simulink model "SEA_system"  (R2023b)
settings: Solver=VariableStepAuto  StartTime=0.0  StopTime=10  FixedStep=0.005  RelTol=1e-3
values from neighbouring files (symbols this model uses):
  c1 = 0.6    [SEA_system.m]
  c2 = 0.6    [SEA_system.m]
  CoM1 = 0.117    [SEA_system.m]
  CoM2 = 0.045    [SEA_system.m]
  Fx = 0    [SEA_system.m]
  Fy = 0    [SEA_system.m]
  g = 9.81    [SEA_system.m]
  J1 = m1*L1^2/12 + m1*CoM1^2    (= 0.00579610927083)    [SEA_system.m]
  J2 = m2*L2^2/12 + m2*CoM2^2 + (mEE*(L2-CoM2)^2)    (= 0.00129963166667)    [SEA_system.m]
  k1 = 5.9*10^3    (= 5900)    [SEA_system.m]
  k2 = 5.9*10^3    (= 5900)    [SEA_system.m]
  L1 = 0.20075    [SEA_system.m]
  L2 = 0.149    [SEA_system.m]
  m1 = 0.340    (= 0.34)    [SEA_system.m]
  m2 = 0.140    (= 0.14)    [SEA_system.m]
  N1 = m1*CoM1^2 + J1 + m2*L1^2 + m2*CoM2^2 + J2    (= 0.0176755796875)    [SEA_system.m]
  N2 = m2*L1*CoM2    (= 0.001264725)    [SEA_system.m]
  N3 = m2*CoM2^2 + J2    (= 0.00158313166667)    [SEA_system.m]
  Px = 0.1    [SEA_system.m]
  Py = 0.05    [SEA_system.m]
libraries: simulink_extras x4, slpidlib x3
settings Model: Creator=Master  LastModifiedBy=tpdnr
settings SolverCC: ZeroCrossAlgorithm=Adaptive
settings DebuggingCC: MaskedZcDiagnostic=none  IgnoredZcDiagnostic=none

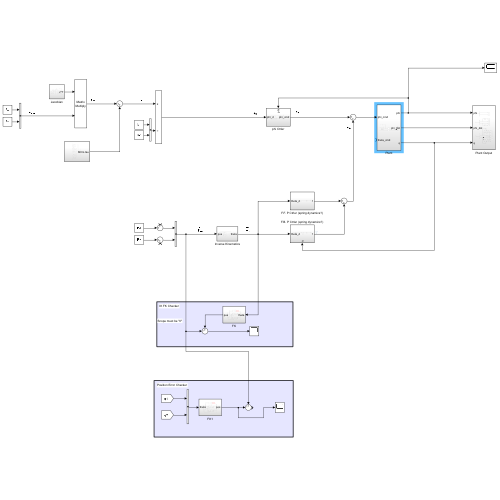
[thumbnail: Simulink's stored preview of the top-level diagram]
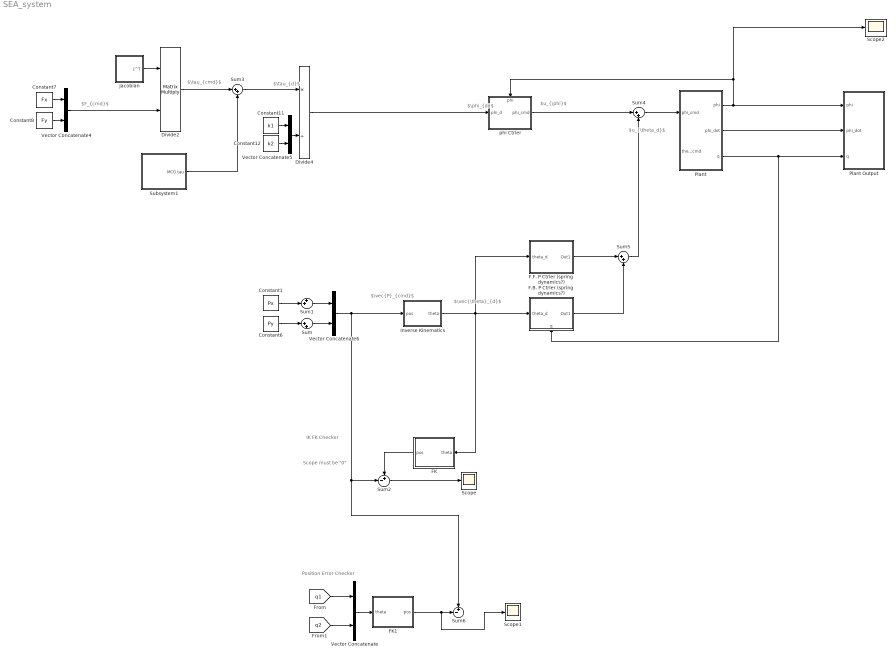
== system SEA_system ==
  note: Position Error Checker
  note: Scope must be "0"
  note: $F_{cmd}$
  note: $\tau_{cmd}$
  note: $\tau_{d}$
  note: $\phi_{d}$
  note: $u_{\phi}$
  note: $\vec{P}_{cmd}$
  note: $\vec{\theta}_{d}$
  note: $u_{\theta_d}$
  note: IK FK Checker
  Constant1 : Constant  Value=Px
  Constant11 : Constant  Value=k1
  Constant12 : Constant  Value=k2
  Constant6 : Constant  Value=Py
  Constant7 : Constant  Value=Fx
  Constant8 : Constant  Value=Fy
  Divide2 : Product  Inputs=**  Multiplication=Matrix(*)
  Divide4 : Product  Inputs=*/
  F.B. P Ctrler (spring dynamics?) : Subsystem
      settings: PortSchema="{\"entries\":[{\"content\":{\"sides\":[{\"content\":{\"connectorIds\":[\"In1\"]},\"type\":\"ConnectorPlacement.EquallySpacedRectSide\",\"uuid\":\"4d208e63-a6c3-42c2-9e85-ad51048c4a51\"},{\"content\":{\"connectorIds\":[\"Out1\"],\"side\":\"RIGHT\"},\"type\":\"ConnectorPlacement.EquallySpacedRectSide\",\"uuid\":\"eee0dd30-27df-41b3-9dcf-f04dc984317a\"},{\"content\":{\"side\":\"TOP\"},\"type\":\"ConnectorPlacement.EquallySpacedRectSide\",\"uuid\":\"b56dc6f1-fbae-4ae5-b685-d1dd5f7423cb\"},{\"content\":{\"connectorIds\":[\"In2\"],\"side\":\"BOTTOM\"},\"type\":\"ConnectorPlacement.EquallySpacedRectSide\",\"uuid\":\"8db1bbe8-a585-485d-a15a-1764a5483703\"}]},\"type\":\"ConnectorPlacement.EquallySpacedConnector\",\"uuid\":\"2ec91dce-e516-4ac5-924e-aa549dba9b81\"}],\"packageUris\":[\"http://schema.mathworks.com/mf0/Connector/R2020b\"],\"version\":\"1.0\"}"
  F.F. P Ctrler (spring dynamics?) : Subsystem
  FK : Subsystem
  FK1 : Subsystem
      settings: PortSchema="{\"entries\":[{\"content\":{\"sides\":[{\"content\":{\"connectorIds\":[\"Out1\"]},\"type\":\"ConnectorPlacement.EquallySpacedRectSide\",\"uuid\":\"9148f4d4-3f7b-4339-b598-70e7eba9c14c\"},{\"content\":{\"connectorIds\":[\"In1\"],\"side\":\"RIGHT\"},\"type\":\"ConnectorPlacement.EquallySpacedRectSide\",\"uuid\":\"2ec983d7-29f9-4bcc-b0b0-e28b197ebcd0\"},{\"content\":{\"side\":\"TOP\"},\"type\":\"ConnectorPlacement.EquallySpacedRectSide\",\"uuid\":\"6d95d5e6-a927-40b0-a022-88fc1901032f\"}]},\"type\":\"ConnectorPlacement.EquallySpacedConnector\",\"uuid\":\"4f8038e9-ada6-4d65-8522-250804851321\"}],\"packageUris\":[\"http://schema.mathworks.com/mf0/Connector/R2020b\"],\"version\":\"1.0\"}"
  Inverse Kinematics : Subsystem
  Jacobian : Subsystem
  Plant : Subsystem
  Plant Output : Subsystem
  Scope : Scope
  Scope1 : Scope
  Scope2 : Scope
  Subsystem1 : Subsystem
  Sum{,3..5} (4 alike) : Sum  Inputs=|++
  Sum1 : Sum  Inputs=++|
  Sum2 : Sum  Inputs=+-|
  Sum6 : Sum  Inputs=+-|
  Vector Concatenate{,4..6} (4 alike) : Concatenate
  phi Ctrler : Subsystem
      settings: PortSchema="{\"entries\":[{\"content\":{\"sides\":[{\"content\":{\"connectorIds\":[\"In1\"]},\"type\":\"ConnectorPlacement.EquallySpacedRectSide\",\"uuid\":\"3d32bdc1-b9b0-4014-9f2c-584152c2ae2a\"},{\"content\":{\"connectorIds\":[\"Out1\"],\"side\":\"RIGHT\"},\"type\":\"ConnectorPlacement.EquallySpacedRectSide\",\"uuid\":\"debc5263-adf8-4ed2-a891-d4f334c5857b\"},{\"content\":{\"connectorIds\":[\"In2\"],\"side\":\"TOP\"},\"type\":\"ConnectorPlacement.EquallySpacedRectSide\",\"uuid\":\"7bd5ab05-8083-45fb-a57a-66a3a725ceed\"}]},\"type\":\"ConnectorPlacement.EquallySpacedConnector\",\"uuid\":\"986cff17-d96f-4d8b-90f2-1c94d4d77448\"}],\"packageUris\":[\"http://schema.mathworks.com/mf0/Connector/R2020b\"],\"version\":\"1.0\"}"
  wires:
  Constant7/1 -> Vector Concatenate4/1
  Constant8/1 -> Vector Concatenate4/2
  Vector Concatenate5/1 -> Divide4/2
  Constant11/1 -> Vector Concatenate5/1
  Constant12/1 -> Vector Concatenate5/2
  Divide4/1 -> phi Ctrler/1(phi_d)
  Inverse Kinematics/1(theta) -> FK/1(theta), F.F. P Ctrler (spring dynamics?)/1(theta_d), F.B. P Ctrler (spring dynamics?)/1(theta_d)
  Plant/1(phi) -> Plant Output/1(phi), phi Ctrler/2(phi), Scope2/1
  Plant/3(q) -> F.B. P Ctrler (spring dynamics?)/2(q), Plant Output/3(q)
  Jacobian/1(J^T) -> Divide2/1
  Vector Concatenate4/1 -> Divide2/2
  Vector Concatenate6/1 -> Sum6/1, Sum2/2, Inverse Kinematics/1(pos)
  Sum5/1 -> Sum4/2
  phi Ctrler/1(phi_cmd) -> Sum4/1
  Constant1/1 -> Sum1/2
  Constant6/1 -> Sum/1
  Sum/1 -> Vector Concatenate6/2
  Sum1/1 -> Vector Concatenate6/1
  FK/1(pos) -> Sum2/1
  [q1] -> Vector Concatenate/1
  [q2] -> Vector Concatenate/2
  Vector Concatenate/1 -> FK1/1(theta)
  F.F. P Ctrler (spring dynamics?)/1(Out1) -> Sum5/1
  F.B. P Ctrler (spring dynamics?)/1(Out1) -> Sum5/2
  Sum2/1 -> Scope/1
  FK1/1(pos) -> Scope1/1, Sum6/2
  Plant/2(phi_dot) -> Plant Output/2(phi_dot)
  Divide2/1 -> Sum3/1
  Subsystem1/1(MCG tau) -> Sum3/2
  Sum3/1 -> Divide4/1
  Sum4/1 -> Plant/1(phi_cmd)

== system SEA_system/F.B. P Ctrler (spring dynamics?) ==
  note: $e_{\theta}$
  note: $Controller$
  theta_d : Inport
  q : Inport  Port=2
  Gain : Gain
  PID Controller : slpidlib/PID Controller  Controller=PID  Form=Parallel  TimeDomain=Continuous-time  UseExternalTs=off  SampleTime=-1  IntegratorMethod=Forward Euler  FilterMethod=Forward Euler  ControllerParametersSource=internal  P=10  I=1  UseKiTs=off  D=0  N=100  UseFilter=on  TunerSelectOption=Transfer Function Based (PID Tuner App)  InitialConditionSource=internal  InitialConditionForIntegrator=0  InitialConditionForFilter=0  DifferentiatorICPrevScaledInput=0  ExternalReset=none  TrackingMode=off  Kt=1  LimitOutput=off  SatLimitsSource=internal  UpperSaturationLimit=inf  LowerSaturationLimit=-inf  LinearizeAsGain=on  AntiWindupMode=none  Kb=1  LimitIntegrator=off  UpperIntegratorSaturationLimit=inf  LowerIntegratorSaturationLimit=-inf  POutMin=[]  POutMax=[]  IOutMin=[]  IOutMax=[]  DOutMin=[]  DOutMax=[]  NOutMin=[]  NOutMax=[]  SumOutMin=[]  SumOutMax=[]  SaturationOutMin=[]  SaturationOutMax=[]  PParamMin=[]  PParamMax=[]  IParamMin=[]  IParamMax=[]  DParamMin=[]  DParamMax=[]  NParamMin=[]  NParamMax=[]  KbParamMin=[]  KbParamMax=[]  KtParamMin=[]  KtParamMax=[]  KbOutMin=[]  KbOutMax=[]  KtOutMin=[]  KtOutMax=[]  IntegratorOutMin=[]  IntegratorOutMax=[]  FilterOutMin=[]  FilterOutMax=[]  SumI1OutMin=[]  SumI1OutMax=[]  SumI2OutMin=[]  SumI2OutMax=[]  SumI3OutMin=[]  SumI3OutMax=[]  SumI4OutMin=[]  SumI4OutMax=[]  SumDOutMin=[]  SumDOutMax=[]  DifferentiatorOutMin=[]  DifferentiatorOutMax=[]  FilterDiffOutCoefMin=[]  FilterDiffOutCoefMax=[]  ReciprocalOutMin=[]  ReciprocalOutMax=[]  SumDenOutMin=[]  SumDenOutMax=[]  SumNumOutMin=[]  SumNumOutMax=[]  DivideOutMin=[]  DivideOutMax=[]  UdiffTsProdOutMin=[]  UdiffTsProdOutMax=[]  NTsProdOutMin=[]  NTsProdOutMax=[]  UintegralTsProdOutMin=[]  UintegralTsProdOutMax=[]  UngainTsProdOutMin=[]  UngainTsProdOutMax=[]  ClampingZeroOutDataTypeStr=Inherit: Inherit via back propagation  ClampingZeroOutMin=[]  ClampingZeroOutMax=[]  FilterDenConstantOutDataTypeStr=Inherit: Inherit via back propagation  FilterDenConstantOutMin=[]  FilterDenConstantOutMax=[]  PCopyOutDataTypeStr=Inherit: Inherit via back propagation  PCopyOutMin=[]  PCopyOutMax=[]  NCopyOutDataTypeStr=Inherit: Inherit via back propagation  NCopyOutMin=[]  NCopyOutMax=[]  IntegratorContinuousStateAttributes=''  IntegratorStateMustResolveToSignalObject=off  IntegratorRTWStateStorageClass=Auto  FilterContinuousStateAttributes=''  FilterStateMustResolveToSignalObject=off  FilterRTWStateStorageClass=Auto  ParallelPVariant=InternalParameters  IdealPVariant=Disabled  IVariant=InternalParameters  DVariant=InternalParameters  IntegratorVariant=Continuous  SatVariant=Disabled  AWVariant=Passthrough  PCopyVariant=Disabled  TRVariant=Disabled  FdbkBlocksVariant=Forward  IdealPFdbkVariant=Disabled  SatFdbkVariant=Disabled  DerivativeFilterVariant=ContFilter  NVariant=InternalParameters  NCopyVariant=Disabled  FilterICVariant=InternalICsFilter  IntegratorICVariant=InternalICs  ExternalResetVariant=Disabled  TRSumVariant=Passthrough  SumFdbkVariant=Disabled  SumVariant=Sum_PID  TsampFilterVariant=InternalTs  TsampNgainVariant=Passthrough  TsampIntegralVariant=Disabled_SignalSpec  ExternalSaturationOutDataTypeStr=Inherit: Same as second input
  Sum : Sum  Inputs=|+-
  Out1 : Outport
  wires:
  Gain/1 -> Out1/1
  theta_d/1 -> Sum/1
  q/1 -> Sum/2
  Sum/1 -> PID Controller/1
  PID Controller/1 -> Gain/1

== system SEA_system/F.F. P Ctrler (spring dynamics?) ==
  note: $Controller$
  theta_d : Inport
  Gain : Gain
  Out1 : Outport
  wires:
  Gain/1 -> Out1/1
  theta_d/1 -> Gain/1

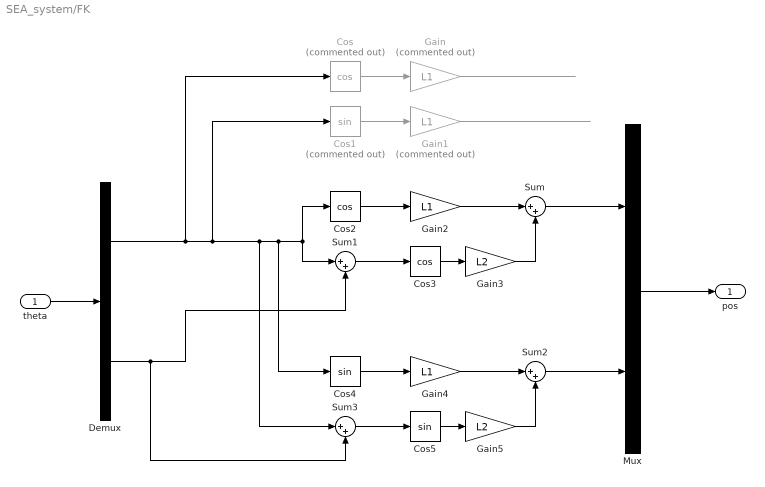
== system SEA_system/FK ==
  theta : Inport
  Cos : Trigonometry  Commented=on  Operator=cos
  Cos1 : Trigonometry  Commented=on
  Cos2 : Trigonometry  Operator=cos
  Cos3 : Trigonometry  Operator=cos
  Cos4 : Trigonometry
  Cos5 : Trigonometry
  Demux : Demux  Outputs=2
  Gain : Gain  Commented=on  Gain=L1
  Gain1 : Gain  Commented=on  Gain=L1
  Gain2 : Gain  Gain=L1
  Gain3 : Gain  Gain=L2
  Gain4 : Gain  Gain=L1
  Gain5 : Gain  Gain=L2
  Mux : Mux  Inputs=2
  Sum{,1..3} (4 alike) : Sum  Inputs=|++
  pos : Outport
  wires:
  Cos2/1 -> Gain2/1
  Cos3/1 -> Gain3/1
  Demux/1 -> Cos/1, Cos1/1, Sum3/1, Cos4/1, Cos2/1, Sum1/1
  Sum/1 -> Mux/1
  Demux/2 -> Sum3/2, Sum1/2
  Cos1/1 -> Gain1/1
  Cos5/1 -> Gain5/1
  Gain2/1 -> Sum/1
  Gain1/1 -> ?
  Cos/1 -> Gain/1
  Sum2/1 -> Mux/2
  Gain4/1 -> Sum2/1
  theta/1 -> Demux/1
  Gain3/1 -> Sum/2
  Sum3/1 -> Cos5/1
  Gain5/1 -> Sum2/2
  Sum1/1 -> Cos3/1
  Cos4/1 -> Gain4/1
  Gain/1 -> ?
  Mux/1 -> pos/1

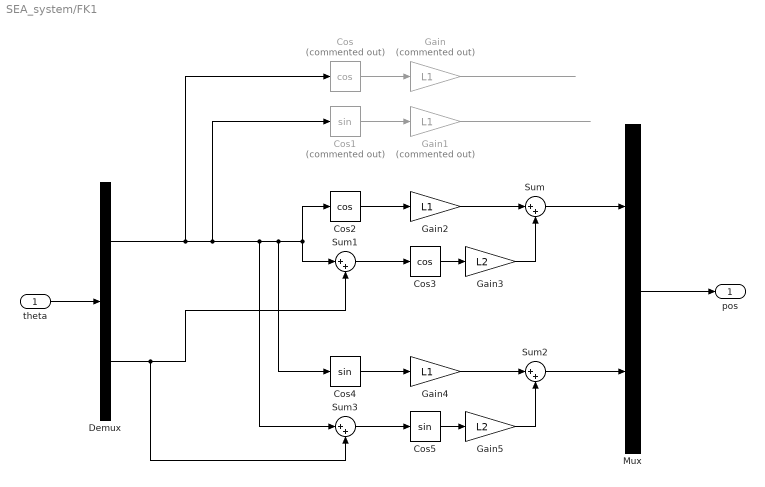
== system SEA_system/FK1 ==
  theta : Inport
  Cos : Trigonometry  Commented=on  Operator=cos
  Cos1 : Trigonometry  Commented=on
  Cos2 : Trigonometry  Operator=cos
  Cos3 : Trigonometry  Operator=cos
  Cos4 : Trigonometry
  Cos5 : Trigonometry
  Demux : Demux  Outputs=2
  Gain : Gain  Commented=on  Gain=L1
  Gain1 : Gain  Commented=on  Gain=L1
  Gain2 : Gain  Gain=L1
  Gain3 : Gain  Gain=L2
  Gain4 : Gain  Gain=L1
  Gain5 : Gain  Gain=L2
  Mux : Mux  Inputs=2
  Sum{,1..3} (4 alike) : Sum  Inputs=|++
  pos : Outport
  wires:
  Cos2/1 -> Gain2/1
  Cos3/1 -> Gain3/1
  Demux/1 -> Cos/1, Cos1/1, Sum3/1, Cos4/1, Cos2/1, Sum1/1
  Sum/1 -> Mux/1
  Demux/2 -> Sum3/2, Sum1/2
  Cos1/1 -> Gain1/1
  Cos5/1 -> Gain5/1
  Gain2/1 -> Sum/1
  Gain1/1 -> ?
  Cos/1 -> Gain/1
  Sum2/1 -> Mux/2
  Gain4/1 -> Sum2/1
  theta/1 -> Demux/1
  Gain3/1 -> Sum/2
  Sum3/1 -> Cos5/1
  Gain5/1 -> Sum2/2
  Sum1/1 -> Cos3/1
  Cos4/1 -> Gain4/1
  Gain/1 -> ?
  Mux/1 -> pos/1

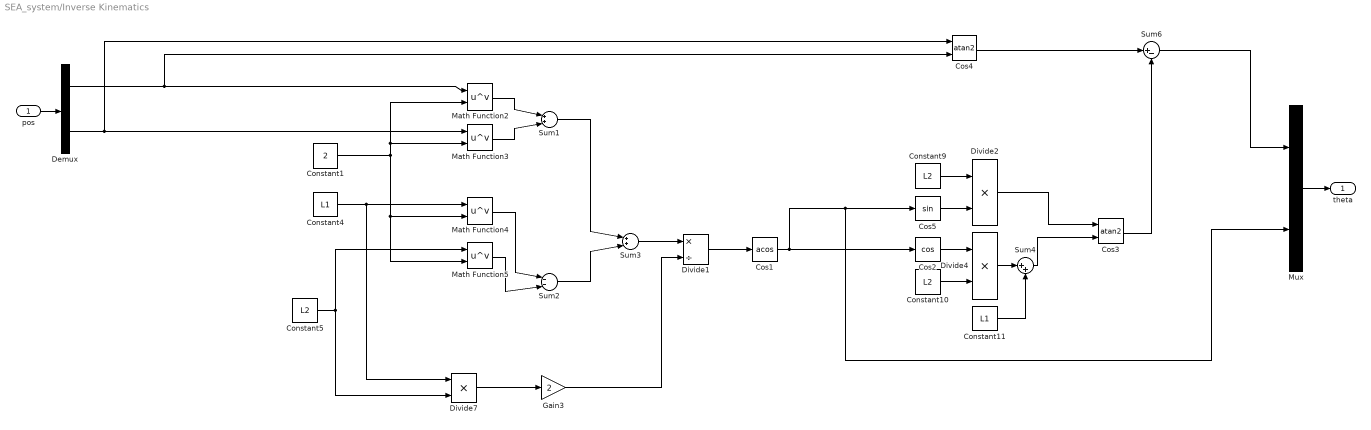
== system SEA_system/Inverse Kinematics ==
  pos : Inport
  Constant1 : Constant  Value=2
  Constant10 : Constant  Value=L2
  Constant11 : Constant  Value=L1
  Constant4 : Constant  Value=L1
  Constant5 : Constant  Value=L2
  Constant9 : Constant  Value=L2
  Cos1 : Trigonometry  Operator=acos
  Cos2 : Trigonometry  Operator=cos
  Cos3 : Trigonometry  Operator=atan2
  Cos4 : Trigonometry  Operator=atan2
  Cos5 : Trigonometry
  Demux : Demux  Outputs=2
  Divide1 : Product  Inputs=*/
  Divide2 : Product  Inputs=**
  Divide4 : Product  Inputs=**
  Divide7 : Product  Inputs=**
  Gain3 : Gain  Gain=2
  Math Function{2..5} (4 alike) : Math  Operator=pow
  Mux : Mux  Inputs=2
  Sum1 : Sum  Inputs=|++|
  Sum2 : Sum  Inputs=|--|
  Sum3 : Sum  Inputs=|++|
  Sum4 : Sum  Inputs=|++
  Sum6 : Sum  Inputs=|+-
  theta : Outport
  wires:
  Sum4/1 -> Cos3/2
  Cos3/1 -> Sum6/2
  Demux/1 -> Cos4/2, Math Function2/1
  Constant1/1 -> Math Function3/2, Math Function2/2, Math Function5/2, Math Function4/2
  Sum3/1 -> Divide1/1
  Constant5/1 -> Math Function5/1, Divide7/2
  Math Function4/1 -> Sum2/1
  Demux/2 -> Cos4/1, Math Function3/1
  Constant4/1 -> Divide7/1, Math Function4/1
  Gain3/1 -> Divide1/2
  Cos1/1 -> Mux/2, Cos5/1, Cos2/1
  Math Function3/1 -> Sum1/2
  Cos5/1 -> Divide2/2
  Constant10/1 -> Divide4/2
  Divide1/1 -> Cos1/1
  Sum1/1 -> Sum3/1
  Constant11/1 -> Sum4/2
  Math Function2/1 -> Sum1/1
  Constant9/1 -> Divide2/1
  Math Function5/1 -> Sum2/2
  Cos2/1 -> Divide4/1
  Cos4/1 -> Sum6/1
  Sum2/1 -> Sum3/2
  Divide7/1 -> Gain3/1
  Divide4/1 -> Sum4/1
  pos/1 -> Demux/1
  Mux/1 -> theta/1
  Divide2/1 -> Cos3/1
  Sum6/1 -> Mux/1

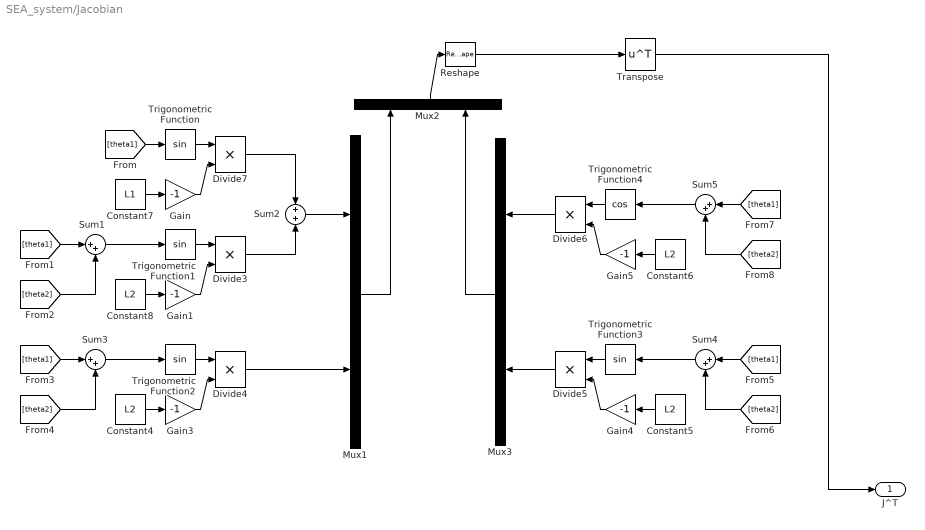
== system SEA_system/Jacobian ==
  Constant{4..6,8} (4 alike) : Constant  Value=L2
  Constant7 : Constant  Value=L1
  Divide{3..7} (5 alike) : Product  Inputs=**
  Gain{,1,3..5} (5 alike) : Gain  Gain=-1
  Mux1 : Mux  Inputs=2
  Mux2 : Mux  Inputs=2
  Mux3 : Mux  Inputs=2
  Reshape : Reshape  OutputDimensionality=Customize  OutputDimensions=[2,2]
  Sum{1,3..5} (4 alike) : Sum  Inputs=|++
  Sum2 : Sum  Inputs=+|+
  Transpose : Math  Operator=transpose
  Trigonometric Function{,1..3} (4 alike) : Trigonometry
  Trigonometric Function4 : Trigonometry  Operator=cos
  J^T : Outport
  wires:
  Gain1/1 -> Divide3/2
  [theta1] -> Sum5/1
  [theta1] -> Trigonometric Function/1
  Trigonometric Function4/1 -> Divide6/1
  Constant8/1 -> Gain1/1
  Mux2/1 -> Reshape/1
  Gain/1 -> Divide7/2
  [theta1] -> Sum4/1
  Constant5/1 -> Gain4/1
  [theta2] -> Sum1/2
  Sum4/1 -> Trigonometric Function3/1
  [theta2] -> Sum5/2
  Constant4/1 -> Gain3/1
  Trigonometric Function2/1 -> Divide4/1
  Divide3/1 -> Sum2/2
  Gain3/1 -> Divide4/2
  Mux1/1 -> Mux2/1
  Gain5/1 -> Divide6/2
  Trigonometric Function/1 -> Divide7/1
  Divide7/1 -> Sum2/1
  Trigonometric Function3/1 -> Divide5/1
  Sum3/1 -> Trigonometric Function2/1
  Sum5/1 -> Trigonometric Function4/1
  Trigonometric Function1/1 -> Divide3/1
  [theta1] -> Sum1/1
  Constant6/1 -> Gain5/1
  [theta2] -> Sum4/2
  Constant7/1 -> Gain/1
  Divide6/1 -> Mux3/1
  Mux3/1 -> Mux2/2
  [theta1] -> Sum3/1
  [theta2] -> Sum3/2
  Sum2/1 -> Mux1/1
  Sum1/1 -> Trigonometric Function1/1
  Gain4/1 -> Divide5/2
  Divide4/1 -> Mux1/2
  Divide5/1 -> Mux3/2
  Reshape/1 -> Transpose/1
  Transpose/1 -> J^T/1

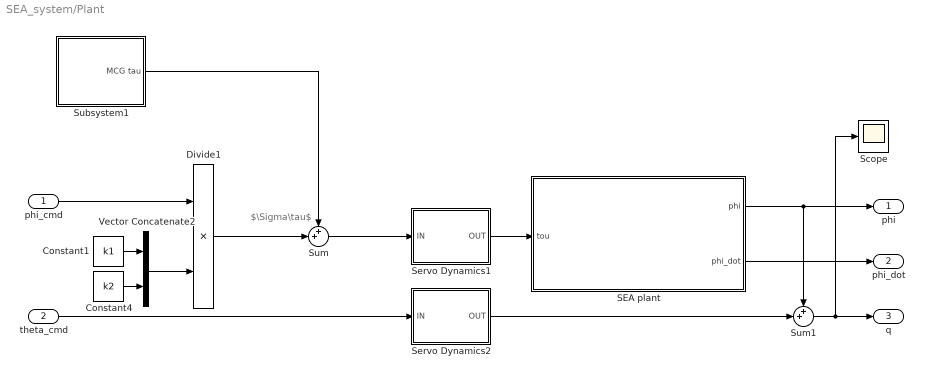
== system SEA_system/Plant ==
  note: $\Sigma\tau$
  phi_cmd : Inport
  theta_cmd : Inport  Port=2
  Constant1 : Constant  Value=k1
  Constant4 : Constant  Value=k2
  Divide1 : Product  Inputs=**
  SEA plant : Subsystem
  Scope : Scope
  Servo Dynamics1 : Subsystem
  Servo Dynamics2 : Subsystem
  Subsystem1 : Subsystem
  Sum : Sum  Inputs=++|
  Sum1 : Sum  Inputs=++|
  Vector Concatenate2 : Concatenate
  phi : Outport
  phi_dot : Outport  Port=2
  q : Outport  Port=3
  wires:
  SEA plant/1(phi) -> Sum1/1, phi/1
  Sum1/1 -> Scope/1, q/1
  Constant4/1 -> Vector Concatenate2/2
  Constant1/1 -> Vector Concatenate2/1
  Vector Concatenate2/1 -> Divide1/2
  phi_cmd/1 -> Divide1/1
  Servo Dynamics2/1(OUT) -> Sum1/2
  Servo Dynamics1/1(OUT) -> SEA plant/1(tou)
  SEA plant/2(phi_dot) -> phi_dot/1
  Subsystem1/1(MCG tau) -> Sum/1
  Sum/1 -> Servo Dynamics1/1(IN)
  theta_cmd/1 -> Servo Dynamics2/1(IN)
  Divide1/1 -> Sum/2

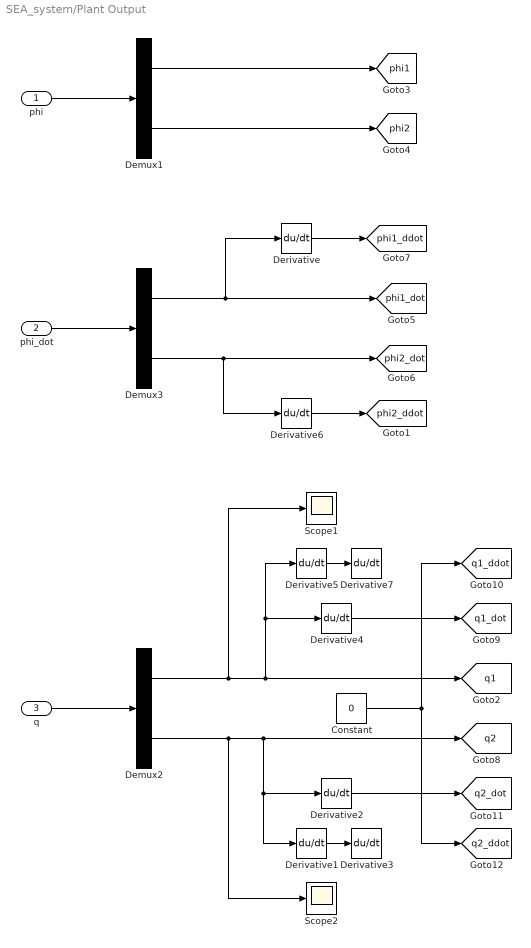
== system SEA_system/Plant Output ==
  phi : Inport
  phi_dot : Inport  Port=2
  q : Inport  Port=3
  Constant : Constant  Value=0
  Demux1 : Demux  Outputs=2
  Demux2 : Demux  Outputs=2
  Demux3 : Demux  Outputs=2
  Derivative{,1..7} (8 alike) : Derivative
  Scope1 : Scope
  Scope2 : Scope
  tag scope: phi1=global, phi1_ddot=global, phi1_dot=global, phi2=global, phi2_ddot=global, phi2_dot=global, q1=global, q1_ddot=global, q1_dot=global, q2=global, q2_ddot=global, q2_dot=global
  wires:
  phi/1 -> Demux1/1
  q/1 -> Demux2/1
  phi_dot/1 -> Demux3/1
  Demux1/2 -> [phi2]
  Demux1/1 -> [phi1]
  Demux3/2 -> Derivative6/1, [phi2_dot]
  Demux3/1 -> Derivative/1, [phi1_dot]
  Derivative/1 -> [phi1_ddot]
  Derivative6/1 -> [phi2_ddot]
  Demux2/1 -> Scope1/1, Derivative5/1, Derivative4/1, [q1]
  Derivative1/1 -> Derivative3/1
  Derivative5/1 -> Derivative7/1
  Demux2/2 -> Derivative1/1, Derivative2/1, [q2], Scope2/1
  Constant/1 -> [q1_ddot], [q2_ddot]
  Derivative4/1 -> [q1_dot]
  Derivative2/1 -> [q2_dot]

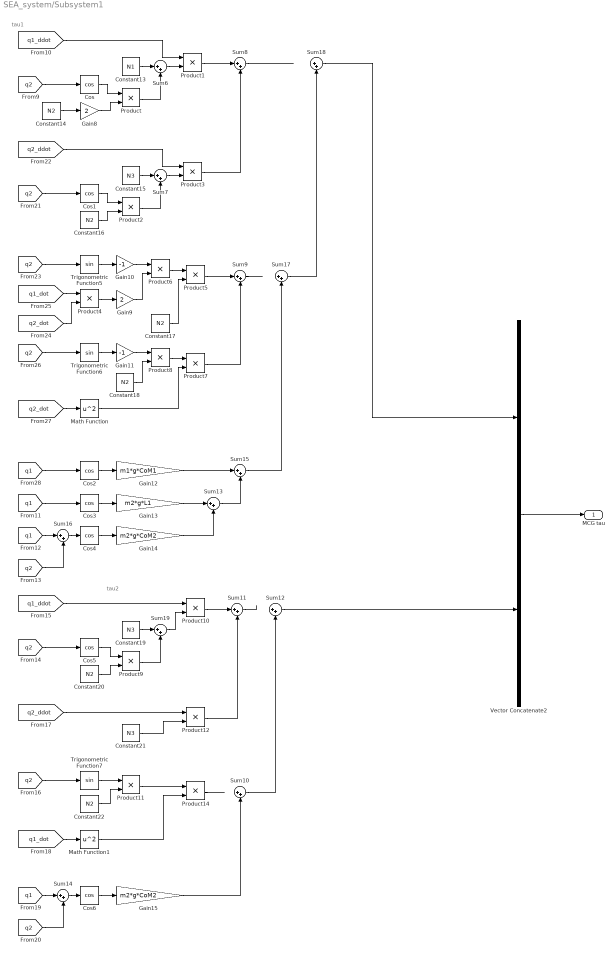
== system SEA_system/Subsystem1 ==
  note: tau2
  note: tau1
  Constant13 : Constant  Value=N1
  Constant{14,16..18,20,22} (6 alike) : Constant  Value=N2
  Constant15 : Constant  Value=N3
  Constant19 : Constant  Value=N3
  Constant21 : Constant  Value=N3
  Cos{,1..6} (7 alike) : Trigonometry  Operator=cos
  Gain10 : Gain  Gain=-1
  Gain11 : Gain  Gain=-1
  Gain12 : Gain  Gain=m1*g*CoM1
  Gain13 : Gain  Gain=m2*g*L1
  Gain14 : Gain  Gain=m2*g*CoM2
  Gain15 : Gain  Gain=m2*g*CoM2
  Gain8 : Gain  Gain=2
  Gain9 : Gain  Gain=2
  Math Function : Math  Operator=square
  Math Function1 : Math  Operator=square
  Product{,1..12,14} (14 alike) : Product
  Sum{6..19} (14 alike) : Sum  Inputs=|++
  Trigonometric Function5 : Trigonometry
  Trigonometric Function6 : Trigonometry
  Trigonometric Function7 : Trigonometry
  Vector Concatenate2 : Concatenate
  MCG tau : Outport
  wires:
  Cos5/1 -> Product9/1
  Constant21/1 -> Product12/2
  Product10/1 -> Sum11/1
  [q1_ddot] -> Product10/1
  Sum11/1 -> ?
  Product12/1 -> Sum11/2
  [q1] -> Sum14/1
  Sum14/1 -> Cos6/1
  Sum10/1 -> Sum12/2
  Product9/1 -> Sum19/2
  Cos6/1 -> Gain15/1
  [q2] -> Sum14/2
  Gain15/1 -> Sum10/2
  [q1_dot] -> Math Function1/1
  Math Function1/1 -> Product14/2
  Constant20/1 -> Product9/2
  [q2_ddot] -> Product12/1
  [q2] -> Cos5/1
  Product11/1 -> Product14/1
  [q2] -> Trigonometric Function7/1
  Trigonometric Function7/1 -> Product11/1
  Constant22/1 -> Product11/2
  Constant19/1 -> Sum19/1
  Product14/1 -> ?
  Sum19/1 -> Product10/2
  Constant17/1 -> Product5/2
  Constant14/1 -> Gain8/1
  Cos4/1 -> Gain14/1
  Product7/1 -> Sum9/2
  Sum17/1 -> Sum18/2
  [q2_dot] -> Math Function/1
  [q1] -> Cos3/1
  Cos/1 -> Product/1
  Product4/1 -> Gain9/1
  Product8/1 -> Product7/1
  [q1_dot] -> Product4/1
  Gain10/1 -> Product6/1
  Constant15/1 -> Sum7/1
  Sum8/1 -> ?
  Math Function/1 -> Product7/2
  Cos3/1 -> Gain13/1
  Gain12/1 -> Sum15/1
  Sum16/1 -> Cos4/1
  [q1] -> Cos2/1
  Product1/1 -> Sum8/1
  [q2] -> Sum16/2
  [q1] -> Sum16/1
  [q2] -> Trigonometric Function6/1
  Product5/1 -> Sum9/1
  Sum13/1 -> Sum15/2
  [q2_dot] -> Product4/2
  Trigonometric Function5/1 -> Gain10/1
  Product/1 -> Sum6/2
  Gain11/1 -> Product8/1
  Sum6/1 -> Product1/2
  Product6/1 -> Product5/1
  Sum9/1 -> ?
  Gain9/1 -> Product6/2
  Trigonometric Function6/1 -> Gain11/1
  Product3/1 -> Sum8/2
  Gain8/1 -> Product/2
  Constant16/1 -> Product2/2
  Constant18/1 -> Product8/2
  Cos1/1 -> Product2/1
  Cos2/1 -> Gain12/1
  Constant13/1 -> Sum6/1
  [q2] -> Cos1/1
  Sum7/1 -> Product3/2
  Gain14/1 -> Sum13/2
  Product2/1 -> Sum7/2
  [q2] -> Trigonometric Function5/1
  [q2_ddot] -> Product3/1
  Sum15/1 -> Sum17/2
  [q2] -> Cos/1
  Gain13/1 -> Sum13/1
  [q1_ddot] -> Product1/1
  Sum18/1 -> Vector Concatenate2/1
  Sum12/1 -> Vector Concatenate2/2
  Vector Concatenate2/1 -> MCG tau/1

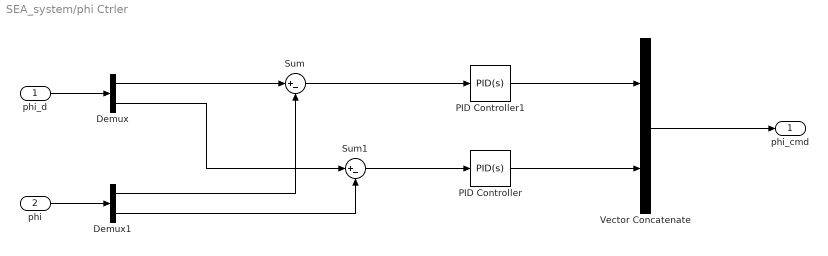
== system SEA_system/phi Ctrler ==
  phi_d : Inport
  phi : Inport  Port=2
  Demux : Demux  Outputs=2
  Demux1 : Demux  Outputs=2
  PID Controller : slpidlib/PID Controller  Controller=PID  Form=Parallel  TimeDomain=Continuous-time  UseExternalTs=off  SampleTime=-1  IntegratorMethod=Forward Euler  FilterMethod=Forward Euler  ControllerParametersSource=internal  P=1  I=0.1  UseKiTs=off  D=0  N=100  UseFilter=on  TunerSelectOption=Transfer Function Based (PID Tuner App)  InitialConditionSource=internal  InitialConditionForIntegrator=0  InitialConditionForFilter=0  DifferentiatorICPrevScaledInput=0  ExternalReset=none  TrackingMode=off  Kt=1  LimitOutput=off  SatLimitsSource=internal  UpperSaturationLimit=inf  LowerSaturationLimit=-inf  LinearizeAsGain=on  AntiWindupMode=none  Kb=1  LimitIntegrator=off  UpperIntegratorSaturationLimit=inf  LowerIntegratorSaturationLimit=-inf  POutMin=[]  POutMax=[]  IOutMin=[]  IOutMax=[]  DOutMin=[]  DOutMax=[]  NOutMin=[]  NOutMax=[]  SumOutMin=[]  SumOutMax=[]  SaturationOutMin=[]  SaturationOutMax=[]  PParamMin=[]  PParamMax=[]  IParamMin=[]  IParamMax=[]  DParamMin=[]  DParamMax=[]  NParamMin=[]  NParamMax=[]  KbParamMin=[]  KbParamMax=[]  KtParamMin=[]  KtParamMax=[]  KbOutMin=[]  KbOutMax=[]  KtOutMin=[]  KtOutMax=[]  IntegratorOutMin=[]  IntegratorOutMax=[]  FilterOutMin=[]  FilterOutMax=[]  SumI1OutMin=[]  SumI1OutMax=[]  SumI2OutMin=[]  SumI2OutMax=[]  SumI3OutMin=[]  SumI3OutMax=[]  SumI4OutMin=[]  SumI4OutMax=[]  SumDOutMin=[]  SumDOutMax=[]  DifferentiatorOutMin=[]  DifferentiatorOutMax=[]  FilterDiffOutCoefMin=[]  FilterDiffOutCoefMax=[]  ReciprocalOutMin=[]  ReciprocalOutMax=[]  SumDenOutMin=[]  SumDenOutMax=[]  SumNumOutMin=[]  SumNumOutMax=[]  DivideOutMin=[]  DivideOutMax=[]  UdiffTsProdOutMin=[]  UdiffTsProdOutMax=[]  NTsProdOutMin=[]  NTsProdOutMax=[]  UintegralTsProdOutMin=[]  UintegralTsProdOutMax=[]  UngainTsProdOutMin=[]  UngainTsProdOutMax=[]  ClampingZeroOutDataTypeStr=Inherit: Inherit via back propagation  ClampingZeroOutMin=[]  ClampingZeroOutMax=[]  FilterDenConstantOutDataTypeStr=Inherit: Inherit via back propagation  FilterDenConstantOutMin=[]  FilterDenConstantOutMax=[]  PCopyOutDataTypeStr=Inherit: Inherit via back propagation  PCopyOutMin=[]  PCopyOutMax=[]  NCopyOutDataTypeStr=Inherit: Inherit via back propagation  NCopyOutMin=[]  NCopyOutMax=[]  IntegratorContinuousStateAttributes=''  IntegratorStateMustResolveToSignalObject=off  IntegratorRTWStateStorageClass=Auto  FilterContinuousStateAttributes=''  FilterStateMustResolveToSignalObject=off  FilterRTWStateStorageClass=Auto  ParallelPVariant=InternalParameters  IdealPVariant=Disabled  IVariant=InternalParameters  DVariant=InternalParameters  IntegratorVariant=Continuous  SatVariant=Disabled  AWVariant=Passthrough  PCopyVariant=Disabled  TRVariant=Disabled  FdbkBlocksVariant=Forward  IdealPFdbkVariant=Disabled  SatFdbkVariant=Disabled  DerivativeFilterVariant=ContFilter  NVariant=InternalParameters  NCopyVariant=Disabled  FilterICVariant=InternalICsFilter  IntegratorICVariant=InternalICs  ExternalResetVariant=Disabled  TRSumVariant=Passthrough  SumFdbkVariant=Disabled  SumVariant=Sum_PID  TsampFilterVariant=InternalTs  TsampNgainVariant=Passthrough  TsampIntegralVariant=Disabled_SignalSpec  ExternalSaturationOutDataTypeStr=Inherit: Same as second input
  PID Controller1 : slpidlib/PID Controller  Controller=PID  Form=Parallel  TimeDomain=Continuous-time  UseExternalTs=off  SampleTime=-1  IntegratorMethod=Forward Euler  FilterMethod=Forward Euler  ControllerParametersSource=internal  P=1  I=0.1  UseKiTs=off  D=0  N=100  UseFilter=on  TunerSelectOption=Transfer Function Based (PID Tuner App)  InitialConditionSource=internal  InitialConditionForIntegrator=0  InitialConditionForFilter=0  DifferentiatorICPrevScaledInput=0  ExternalReset=none  TrackingMode=off  Kt=1  LimitOutput=off  SatLimitsSource=internal  UpperSaturationLimit=inf  LowerSaturationLimit=-inf  LinearizeAsGain=on  AntiWindupMode=none  Kb=1  LimitIntegrator=off  UpperIntegratorSaturationLimit=inf  LowerIntegratorSaturationLimit=-inf  POutMin=[]  POutMax=[]  IOutMin=[]  IOutMax=[]  DOutMin=[]  DOutMax=[]  NOutMin=[]  NOutMax=[]  SumOutMin=[]  SumOutMax=[]  SaturationOutMin=[]  SaturationOutMax=[]  PParamMin=[]  PParamMax=[]  IParamMin=[]  IParamMax=[]  DParamMin=[]  DParamMax=[]  NParamMin=[]  NParamMax=[]  KbParamMin=[]  KbParamMax=[]  KtParamMin=[]  KtParamMax=[]  KbOutMin=[]  KbOutMax=[]  KtOutMin=[]  KtOutMax=[]  IntegratorOutMin=[]  IntegratorOutMax=[]  FilterOutMin=[]  FilterOutMax=[]  SumI1OutMin=[]  SumI1OutMax=[]  SumI2OutMin=[]  SumI2OutMax=[]  SumI3OutMin=[]  SumI3OutMax=[]  SumI4OutMin=[]  SumI4OutMax=[]  SumDOutMin=[]  SumDOutMax=[]  DifferentiatorOutMin=[]  DifferentiatorOutMax=[]  FilterDiffOutCoefMin=[]  FilterDiffOutCoefMax=[]  ReciprocalOutMin=[]  ReciprocalOutMax=[]  SumDenOutMin=[]  SumDenOutMax=[]  SumNumOutMin=[]  SumNumOutMax=[]  DivideOutMin=[]  DivideOutMax=[]  UdiffTsProdOutMin=[]  UdiffTsProdOutMax=[]  NTsProdOutMin=[]  NTsProdOutMax=[]  UintegralTsProdOutMin=[]  UintegralTsProdOutMax=[]  UngainTsProdOutMin=[]  UngainTsProdOutMax=[]  ClampingZeroOutDataTypeStr=Inherit: Inherit via back propagation  ClampingZeroOutMin=[]  ClampingZeroOutMax=[]  FilterDenConstantOutDataTypeStr=Inherit: Inherit via back propagation  FilterDenConstantOutMin=[]  FilterDenConstantOutMax=[]  PCopyOutDataTypeStr=Inherit: Inherit via back propagation  PCopyOutMin=[]  PCopyOutMax=[]  NCopyOutDataTypeStr=Inherit: Inherit via back propagation  NCopyOutMin=[]  NCopyOutMax=[]  IntegratorContinuousStateAttributes=''  IntegratorStateMustResolveToSignalObject=off  IntegratorRTWStateStorageClass=Auto  FilterContinuousStateAttributes=''  FilterStateMustResolveToSignalObject=off  FilterRTWStateStorageClass=Auto  ParallelPVariant=InternalParameters  IdealPVariant=Disabled  IVariant=InternalParameters  DVariant=InternalParameters  IntegratorVariant=Continuous  SatVariant=Disabled  AWVariant=Passthrough  PCopyVariant=Disabled  TRVariant=Disabled  FdbkBlocksVariant=Forward  IdealPFdbkVariant=Disabled  SatFdbkVariant=Disabled  DerivativeFilterVariant=ContFilter  NVariant=InternalParameters  NCopyVariant=Disabled  FilterICVariant=InternalICsFilter  IntegratorICVariant=InternalICs  ExternalResetVariant=Disabled  TRSumVariant=Passthrough  SumFdbkVariant=Disabled  SumVariant=Sum_PID  TsampFilterVariant=InternalTs  TsampNgainVariant=Passthrough  TsampIntegralVariant=Disabled_SignalSpec  ExternalSaturationOutDataTypeStr=Inherit: Same as second input
  Sum : Sum  Inputs=|+-
  Sum1 : Sum  Inputs=|+-
  Vector Concatenate : Concatenate
  phi_cmd : Outport
  wires:
  phi_d/1 -> Demux/1
  phi/1 -> Demux1/1
  Demux/1 -> Sum/1
  Demux/2 -> Sum1/1
  PID Controller1/1 -> Vector Concatenate/1
  Vector Concatenate/1 -> phi_cmd/1
  Demux1/1 -> Sum/2
  Demux1/2 -> Sum1/2
  PID Controller/1 -> Vector Concatenate/2
  Sum/1 -> PID Controller1/1
  Sum1/1 -> PID Controller/1

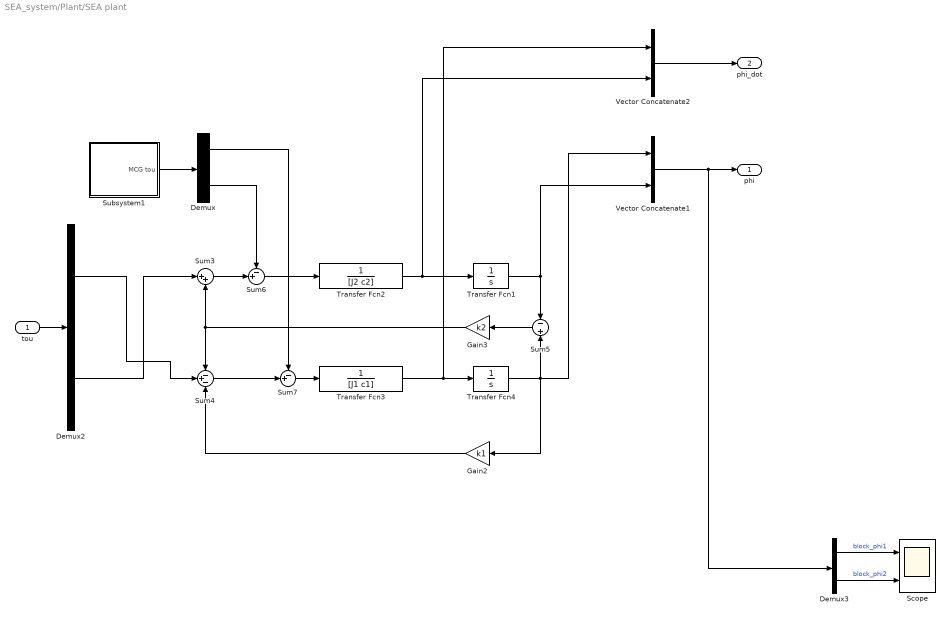
== system SEA_system/Plant/SEA plant ==
  tou : Inport
  Demux : Demux  Outputs=2
  Demux2 : Demux  Outputs=2
  Demux3 : Demux  Outputs=2
  Gain2 : Gain  Gain=k1
  Gain3 : Gain  Gain=k2
  Scope : Scope  NumInputPorts=2
  Subsystem1 : Subsystem
  Sum3 : Sum  Inputs=|++
  Sum4 : Sum  Inputs=-+-
  Sum5 : Sum  Inputs=-|+
  Sum6 : Sum  Inputs=-+|
  Sum7 : Sum  Inputs=-+|
  Transfer Fcn1 : TransferFcn  Denominator=[1 0]
  Transfer Fcn2 : TransferFcn  Denominator=[J2 c2]
  Transfer Fcn3 : TransferFcn  Denominator=[J1 c1]
  Transfer Fcn4 : TransferFcn  Denominator=[1 0]
  Vector Concatenate1 : Concatenate
  Vector Concatenate2 : Concatenate
  phi : Outport
  phi_dot : Outport  Port=2
  wires:
  Subsystem1/1(MCG tou) -> Demux/1
  Transfer Fcn3/1 -> Vector Concatenate2/1, Transfer Fcn4/1
  Gain3/1 -> Sum3/2, Sum4/1
  Sum6/1 -> Transfer Fcn2/1
  Transfer Fcn2/1 -> Vector Concatenate2/2, Transfer Fcn1/1
  Sum5/1 -> Gain3/1
  Vector Concatenate1/1 -> Demux3/1, phi/1
  Sum7/1 -> Transfer Fcn3/1
  Gain2/1 -> Sum4/3
  Demux/2 -> Sum6/1
  Demux2/2 -> Sum3/1
  Demux/1 -> Sum7/1
  Demux2/1 -> Sum4/2
  Sum4/1 -> Sum7/2
  tou/1 -> Demux2/1
  Transfer Fcn1/1 -> Sum5/1, Vector Concatenate1/2
  Transfer Fcn4/1 -> Gain2/1, Vector Concatenate1/1, Sum5/2
  Vector Concatenate2/1 -> phi_dot/1
  Demux3/1 -> Scope/1  "block_phi1"
  Demux3/2 -> Scope/2  "block_phi2"
  Sum3/1 -> Sum6/2

== system SEA_system/Plant/Servo Dynamics1 ==
  IN : Inport
  Demux1 : Demux  Outputs=2
  Mux4 : Mux  Inputs=2
  Saturation{1..2,7..8} (4 alike) : Saturate  UpperLimit=5  LowerLimit=-5
  Servo 1 Dynamics : simulink_extras/Additional Linear/Transfer Fcn (with initial outputs)  N=[1]  D="[1/10  1]"  Y0=0  U0=0
  Servo 2 Dynamics : simulink_extras/Additional Linear/Transfer Fcn (with initial outputs)  N=[1]  D="[1/10  1]"  Y0=0  U0=0
  OUT : Outport
  wires:
  Saturation2/1 -> Mux4/2  "theta_2"
  Saturation1/1 -> Mux4/1  "theta_1"
  Saturation8/1 -> Servo 2 Dynamics/1
  Demux1/1 -> Saturation7/1
  Demux1/2 -> Saturation8/1
  Saturation7/1 -> Servo 1 Dynamics/1
  Servo 2 Dynamics/1 -> Saturation2/1
  Servo 1 Dynamics/1 -> Saturation1/1
  IN/1 -> Demux1/1
  Mux4/1 -> OUT/1

== system SEA_system/Plant/Servo Dynamics2 ==
  IN : Inport
  Demux1 : Demux  Outputs=2
  Mux4 : Mux  Inputs=2
  Saturation{1..2,7..8} (4 alike) : Saturate  UpperLimit=0.3  LowerLimit=-0.3
  Servo 1 Dynamics : simulink_extras/Additional Linear/Transfer Fcn (with initial outputs)  N=[1]  D="[1/10  1]"  Y0=0  U0=0
  Servo 2 Dynamics : simulink_extras/Additional Linear/Transfer Fcn (with initial outputs)  N=[1]  D="[1/10  1]"  Y0=0  U0=0
  OUT : Outport
  wires:
  Saturation2/1 -> Mux4/2  "theta_2"
  Saturation1/1 -> Mux4/1  "theta_1"
  Saturation8/1 -> Servo 2 Dynamics/1
  Demux1/1 -> Saturation7/1
  Demux1/2 -> Saturation8/1
  Saturation7/1 -> Servo 1 Dynamics/1
  Servo 2 Dynamics/1 -> Saturation2/1
  Servo 1 Dynamics/1 -> Saturation1/1
  IN/1 -> Demux1/1
  Mux4/1 -> OUT/1

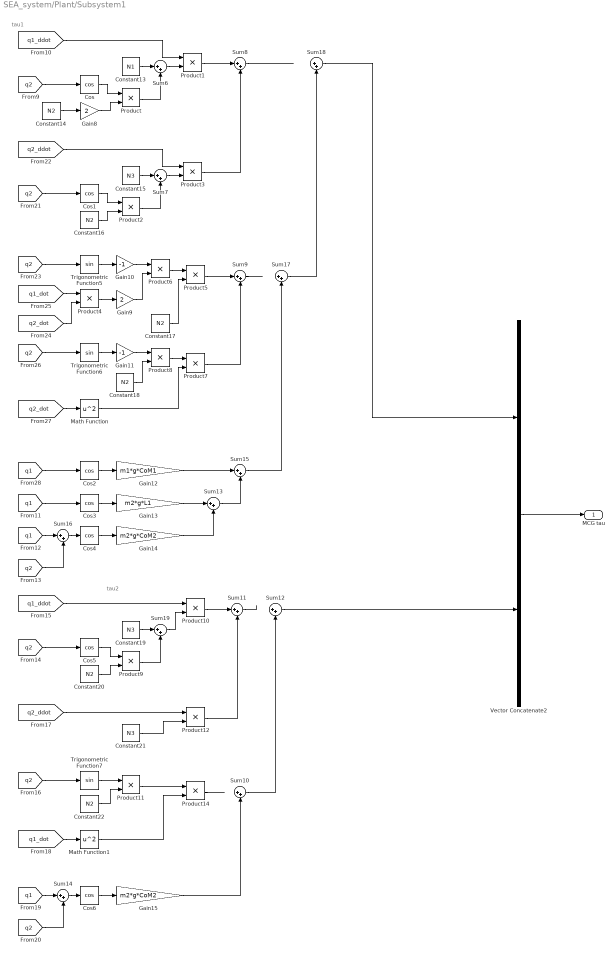
== system SEA_system/Plant/Subsystem1 ==
  note: tau2
  note: tau1
  Constant13 : Constant  Value=N1
  Constant{14,16..18,20,22} (6 alike) : Constant  Value=N2
  Constant15 : Constant  Value=N3
  Constant19 : Constant  Value=N3
  Constant21 : Constant  Value=N3
  Cos{,1..6} (7 alike) : Trigonometry  Operator=cos
  Gain10 : Gain  Gain=-1
  Gain11 : Gain  Gain=-1
  Gain12 : Gain  Gain=m1*g*CoM1
  Gain13 : Gain  Gain=m2*g*L1
  Gain14 : Gain  Gain=m2*g*CoM2
  Gain15 : Gain  Gain=m2*g*CoM2
  Gain8 : Gain  Gain=2
  Gain9 : Gain  Gain=2
  Math Function : Math  Operator=square
  Math Function1 : Math  Operator=square
  Product{,1..12,14} (14 alike) : Product
  Sum{6..19} (14 alike) : Sum  Inputs=|++
  Trigonometric Function5 : Trigonometry
  Trigonometric Function6 : Trigonometry
  Trigonometric Function7 : Trigonometry
  Vector Concatenate2 : Concatenate
  MCG tau : Outport
  wires:
  Cos5/1 -> Product9/1
  Constant21/1 -> Product12/2
  Product10/1 -> Sum11/1
  [q1_ddot] -> Product10/1
  Sum11/1 -> ?
  Product12/1 -> Sum11/2
  [q1] -> Sum14/1
  Sum14/1 -> Cos6/1
  Sum10/1 -> Sum12/2
  Product9/1 -> Sum19/2
  Cos6/1 -> Gain15/1
  [q2] -> Sum14/2
  Gain15/1 -> Sum10/2
  [q1_dot] -> Math Function1/1
  Math Function1/1 -> Product14/2
  Constant20/1 -> Product9/2
  [q2_ddot] -> Product12/1
  [q2] -> Cos5/1
  Product11/1 -> Product14/1
  [q2] -> Trigonometric Function7/1
  Trigonometric Function7/1 -> Product11/1
  Constant22/1 -> Product11/2
  Constant19/1 -> Sum19/1
  Product14/1 -> ?
  Sum19/1 -> Product10/2
  Constant17/1 -> Product5/2
  Constant14/1 -> Gain8/1
  Cos4/1 -> Gain14/1
  Product7/1 -> Sum9/2
  Sum17/1 -> Sum18/2
  [q2_dot] -> Math Function/1
  [q1] -> Cos3/1
  Cos/1 -> Product/1
  Product4/1 -> Gain9/1
  Product8/1 -> Product7/1
  [q1_dot] -> Product4/1
  Gain10/1 -> Product6/1
  Constant15/1 -> Sum7/1
  Sum8/1 -> ?
  Math Function/1 -> Product7/2
  Cos3/1 -> Gain13/1
  Gain12/1 -> Sum15/1
  Sum16/1 -> Cos4/1
  [q1] -> Cos2/1
  Product1/1 -> Sum8/1
  [q2] -> Sum16/2
  [q1] -> Sum16/1
  [q2] -> Trigonometric Function6/1
  Product5/1 -> Sum9/1
  Sum13/1 -> Sum15/2
  [q2_dot] -> Product4/2
  Trigonometric Function5/1 -> Gain10/1
  Product/1 -> Sum6/2
  Gain11/1 -> Product8/1
  Sum6/1 -> Product1/2
  Product6/1 -> Product5/1
  Sum9/1 -> ?
  Gain9/1 -> Product6/2
  Trigonometric Function6/1 -> Gain11/1
  Product3/1 -> Sum8/2
  Gain8/1 -> Product/2
  Constant16/1 -> Product2/2
  Constant18/1 -> Product8/2
  Cos1/1 -> Product2/1
  Cos2/1 -> Gain12/1
  Constant13/1 -> Sum6/1
  [q2] -> Cos1/1
  Sum7/1 -> Product3/2
  Gain14/1 -> Sum13/2
  Product2/1 -> Sum7/2
  [q2] -> Trigonometric Function5/1
  [q2_ddot] -> Product3/1
  Sum15/1 -> Sum17/2
  [q2] -> Cos/1
  Gain13/1 -> Sum13/1
  [q1_ddot] -> Product1/1
  Sum18/1 -> Vector Concatenate2/1
  Sum12/1 -> Vector Concatenate2/2
  Vector Concatenate2/1 -> MCG tau/1

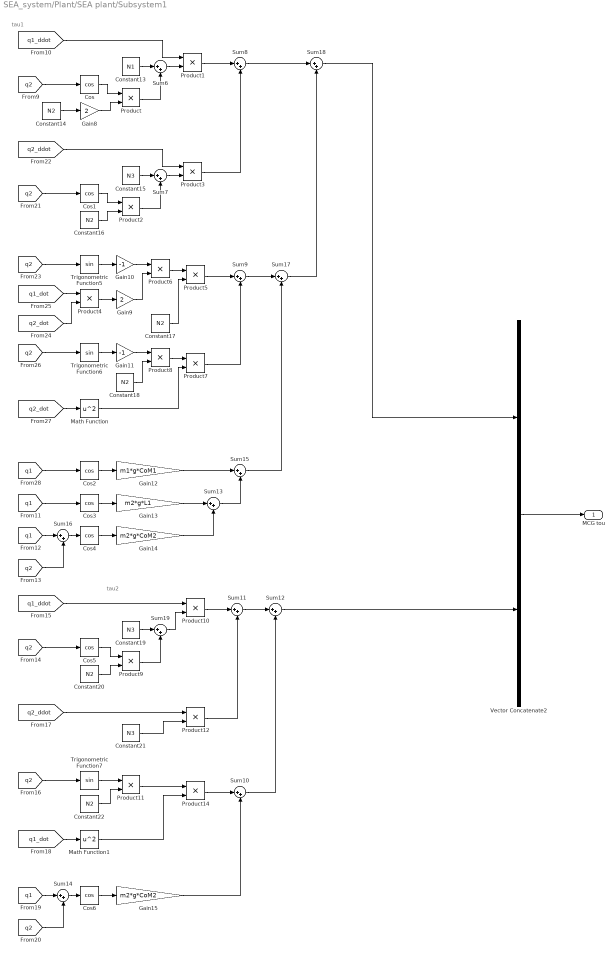
== system SEA_system/Plant/SEA plant/Subsystem1 ==
  note: tau2
  note: tau1
  Constant13 : Constant  Value=N1
  Constant{14,16..18,20,22} (6 alike) : Constant  Value=N2
  Constant15 : Constant  Value=N3
  Constant19 : Constant  Value=N3
  Constant21 : Constant  Value=N3
  Cos{,1..6} (7 alike) : Trigonometry  Operator=cos
  Gain10 : Gain  Gain=-1
  Gain11 : Gain  Gain=-1
  Gain12 : Gain  Gain=m1*g*CoM1
  Gain13 : Gain  Gain=m2*g*L1
  Gain14 : Gain  Gain=m2*g*CoM2
  Gain15 : Gain  Gain=m2*g*CoM2
  Gain8 : Gain  Gain=2
  Gain9 : Gain  Gain=2
  Math Function : Math  Operator=square
  Math Function1 : Math  Operator=square
  Product{,1..12,14} (14 alike) : Product
  Sum{6..19} (14 alike) : Sum  Inputs=|++
  Trigonometric Function5 : Trigonometry
  Trigonometric Function6 : Trigonometry
  Trigonometric Function7 : Trigonometry
  Vector Concatenate2 : Concatenate
  MCG tou : Outport
  wires:
  Cos5/1 -> Product9/1
  Constant21/1 -> Product12/2
  Product10/1 -> Sum11/1
  [q1_ddot] -> Product10/1
  Sum11/1 -> Sum12/1
  Product12/1 -> Sum11/2
  [q1] -> Sum14/1
  Sum14/1 -> Cos6/1
  Sum10/1 -> Sum12/2
  Product9/1 -> Sum19/2
  Cos6/1 -> Gain15/1
  [q2] -> Sum14/2
  Gain15/1 -> Sum10/2
  [q1_dot] -> Math Function1/1
  Math Function1/1 -> Product14/2
  Constant20/1 -> Product9/2
  [q2_ddot] -> Product12/1
  [q2] -> Cos5/1
  Product11/1 -> Product14/1
  [q2] -> Trigonometric Function7/1
  Trigonometric Function7/1 -> Product11/1
  Constant22/1 -> Product11/2
  Constant19/1 -> Sum19/1
  Product14/1 -> Sum10/1
  Sum19/1 -> Product10/2
  Constant17/1 -> Product5/2
  Constant14/1 -> Gain8/1
  Cos4/1 -> Gain14/1
  Product7/1 -> Sum9/2
  Sum17/1 -> Sum18/2
  [q2_dot] -> Math Function/1
  [q1] -> Cos3/1
  Cos/1 -> Product/1
  Product4/1 -> Gain9/1
  Product8/1 -> Product7/1
  [q1_dot] -> Product4/1
  Gain10/1 -> Product6/1
  Constant15/1 -> Sum7/1
  Sum8/1 -> Sum18/1
  Math Function/1 -> Product7/2
  Cos3/1 -> Gain13/1
  Gain12/1 -> Sum15/1
  Sum16/1 -> Cos4/1
  [q1] -> Cos2/1
  Product1/1 -> Sum8/1
  [q2] -> Sum16/2
  [q1] -> Sum16/1
  [q2] -> Trigonometric Function6/1
  Product5/1 -> Sum9/1
  Sum13/1 -> Sum15/2
  [q2_dot] -> Product4/2
  Trigonometric Function5/1 -> Gain10/1
  Product/1 -> Sum6/2
  Gain11/1 -> Product8/1
  Sum6/1 -> Product1/2
  Product6/1 -> Product5/1
  Sum9/1 -> Sum17/1
  Gain9/1 -> Product6/2
  Trigonometric Function6/1 -> Gain11/1
  Product3/1 -> Sum8/2
  Gain8/1 -> Product/2
  Constant16/1 -> Product2/2
  Constant18/1 -> Product8/2
  Cos1/1 -> Product2/1
  Cos2/1 -> Gain12/1
  Constant13/1 -> Sum6/1
  [q2] -> Cos1/1
  Sum7/1 -> Product3/2
  Gain14/1 -> Sum13/2
  Product2/1 -> Sum7/2
  [q2] -> Trigonometric Function5/1
  [q2_ddot] -> Product3/1
  Sum15/1 -> Sum17/2
  [q2] -> Cos/1
  Gain13/1 -> Sum13/1
  [q1_ddot] -> Product1/1
  Sum18/1 -> Vector Concatenate2/1
  Sum12/1 -> Vector Concatenate2/2
  Vector Concatenate2/1 -> MCG tou/1
